simulink model "case2"  (R2024b)
settings: Solver=FixedStepAuto  StartTime=0  StopTime=1  FixedStep=1e-7  RelTol=1e-3
values from neighbouring files (symbols this model uses):
  SG_D_1_D = 0.01056    [IEEE9_case_parameters.m]    (also in case1_parameters.m; case2_parameters.m; case3_parameters.m; case4_parameters.m)
  SG_D_1_EnableSaturation = 0    [IEEE9_case_parameters.m]    (also in case1_parameters.m; case2_parameters.m; case3_parameters.m; case4_parameters.m)
  SG_D_1_f0 = 60    [IEEE9_case_parameters.m]    (also in case1_parameters.m; case2_parameters.m; case3_parameters.m; case4_parameters.m)
  SG_D_1_H = 7.5    [IEEE9_case_parameters.m]    (also in case1_parameters.m; case2_parameters.m; case3_parameters.m; case4_parameters.m)
  SG_D_1_K_A = 20    [IEEE9_case_parameters.m]    (also in case1_parameters.m; case2_parameters.m; case3_parameters.m; case4_parameters.m)
  SG_D_1_K_E = 1.000000e+1    (= 10)    [IEEE9_case_parameters.m]    (also in case1_parameters.m; case2_parameters.m; case3_parameters.m; case4_parameters.m)
  SG_D_1_K_F = 2.363    [IEEE9_case_parameters.m]    (also in case1_parameters.m; case2_parameters.m; case3_parameters.m; case4_parameters.m)
  SG_D_1_K_s = 0.5    [IEEE9_case_parameters.m]    (also in case1_parameters.m = 5; case2_parameters.m = 5; case3_parameters.m = 5; case4_parameters.m = 5)
  SG_D_1_R_a = 0.001088    [IEEE9_case_parameters.m]    (also in case1_parameters.m; case2_parameters.m; case3_parameters.m; case4_parameters.m)
  SG_D_1_S_A = 1    [IEEE9_case_parameters.m]    (also in case1_parameters.m; case2_parameters.m; case3_parameters.m; case4_parameters.m)
  SG_D_1_S_B = 0.103    [IEEE9_case_parameters.m]    (also in case1_parameters.m; case2_parameters.m; case3_parameters.m; case4_parameters.m)
  SG_D_1_S_N = 10.659857    [IEEE9_case_parameters.m]    (also in case1_parameters.m; case2_parameters.m; case3_parameters.m; case4_parameters.m)
  SG_D_1_SpeedPara = 200    [IEEE9_case_parameters.m]    (also in case1_parameters.m; case2_parameters.m; case3_parameters.m; case4_parameters.m)
  SG_D_1_T_0 = 0.720173    [IEEE9_case_parameters.m]    (also in case1_parameters.m = 0.755522; case2_parameters.m = 0.808931; case3_parameters.m = 0.869402; case4_parameters.m = 0.729316)
  SG_D_1_T_1 = 0.3    [IEEE9_case_parameters.m]    (also in case1_parameters.m; case2_parameters.m; case3_parameters.m; case4_parameters.m)
  SG_D_1_T_2 = 0.05    [IEEE9_case_parameters.m]    (also in case1_parameters.m; case2_parameters.m; case3_parameters.m; case4_parameters.m)
  SG_D_1_T_3 = 0.02    [IEEE9_case_parameters.m]    (also in case1_parameters.m; case2_parameters.m; case3_parameters.m; case4_parameters.m)
  SG_D_1_T_4 = 0.005    [IEEE9_case_parameters.m]    (also in case1_parameters.m; case2_parameters.m; case3_parameters.m; case4_parameters.m)
  SG_D_1_T_A = 0.02    [IEEE9_case_parameters.m]    (also in case1_parameters.m; case2_parameters.m; case3_parameters.m; case4_parameters.m)
  SG_D_1_T_dd = 8.000000e+0    (= 8)    [IEEE9_case_parameters.m]    (also in case1_parameters.m; case2_parameters.m; case3_parameters.m; case4_parameters.m)
  SG_D_1_T_ddd = 0.04    [IEEE9_case_parameters.m]    (also in case1_parameters.m; case2_parameters.m; case3_parameters.m; case4_parameters.m)
  SG_D_1_T_E = 0.314    [IEEE9_case_parameters.m]    (also in case1_parameters.m; case2_parameters.m; case3_parameters.m; case4_parameters.m)
  SG_D_1_T_F = 0.35    [IEEE9_case_parameters.m]    (also in case1_parameters.m; case2_parameters.m; case3_parameters.m; case4_parameters.m)
  SG_D_1_T_qd = 0.8    [IEEE9_case_parameters.m]    (also in case1_parameters.m; case2_parameters.m; case3_parameters.m; case4_parameters.m)
  SG_D_1_T_qdd = 0.02    [IEEE9_case_parameters.m]    (also in case1_parameters.m; case2_parameters.m; case3_parameters.m; case4_parameters.m)
  SG_D_1_T_speed = 0.1    [IEEE9_case_parameters.m]    (also in case1_parameters.m = 200; case2_parameters.m = 200; case3_parameters.m = 200; case4_parameters.m = 200)
  SG_D_1_T_w = 0.5    [IEEE9_case_parameters.m]    (also in case1_parameters.m; case2_parameters.m; case3_parameters.m; case4_parameters.m)
  SG_D_1_V_ref = 1.990276    [IEEE9_case_parameters.m]    (also in case1_parameters.m = 2.042296; case2_parameters.m = 2.051388; case3_parameters.m = 2.089584; case4_parameters.m = 2.01845)
  SG_D_1_w_ref = 376.991118    [IEEE9_case_parameters.m]    (also in case1_parameters.m; case2_parameters.m; case3_parameters.m; case4_parameters.m)
  SG_D_1_wb = 6.000000e+1    (= 60)    [IEEE9_case_parameters.m]    (also in case1_parameters.m; case2_parameters.m; case3_parameters.m; case4_parameters.m)
  SG_D_1_x_d = 1.9    [IEEE9_case_parameters.m]    (also in case1_parameters.m; case2_parameters.m; case3_parameters.m; case4_parameters.m)
  SG_D_1_x_dd = 0.302    [IEEE9_case_parameters.m]    (also in case1_parameters.m; case2_parameters.m; case3_parameters.m; case4_parameters.m)
  SG_D_1_x_ddd = 0.204    [IEEE9_case_parameters.m]    (also in case1_parameters.m; case2_parameters.m; case3_parameters.m; case4_parameters.m)
  SG_D_1_x_l = 0.05    [IEEE9_case_parameters.m]    (also in case1_parameters.m; case2_parameters.m; case3_parameters.m; case4_parameters.m)
  SG_D_1_x_q = 1.3    [IEEE9_case_parameters.m]    (also in case1_parameters.m; case2_parameters.m; case3_parameters.m; case4_parameters.m)
  SG_D_1_x_qd = 0.5    [IEEE9_case_parameters.m]    (also in case1_parameters.m; case2_parameters.m; case3_parameters.m; case4_parameters.m)
  SG_D_1_x_qdd = 0.3    [IEEE9_case_parameters.m]    (also in case1_parameters.m; case2_parameters.m; case3_parameters.m; case4_parameters.m)
  SG_D_2_D = 0.02    [IEEE9_case_parameters.m]    (also in case1_parameters.m; case2_parameters.m; case3_parameters.m; case4_parameters.m)
  SG_D_2_EnableSaturation = 0    [IEEE9_case_parameters.m]    (also in case1_parameters.m; case2_parameters.m; case3_parameters.m; case4_parameters.m)
  SG_D_2_f0 = 60    [IEEE9_case_parameters.m]    (also in case1_parameters.m; case2_parameters.m; case3_parameters.m; case4_parameters.m)
  SG_D_2_H = 8.000000e+0    (= 8)    [IEEE9_case_parameters.m]    (also in case1_parameters.m; case2_parameters.m; case3_parameters.m; case4_parameters.m)
  SG_D_2_K_A = 20    [IEEE9_case_parameters.m]    (also in case1_parameters.m; case2_parameters.m; case3_parameters.m; case4_parameters.m)
  SG_D_2_K_E = 1.000000e+1    (= 10)    [IEEE9_case_parameters.m]    (also in case1_parameters.m; case2_parameters.m; case3_parameters.m; case4_parameters.m)
  SG_D_2_K_F = 2.363    [IEEE9_case_parameters.m]    (also in case1_parameters.m; case2_parameters.m; case3_parameters.m; case4_parameters.m)
  SG_D_2_K_s = 0.5    [IEEE9_case_parameters.m]    (also in case1_parameters.m = 4; case2_parameters.m = 4; case3_parameters.m = 4; case4_parameters.m = 4)
  SG_D_2_R_a = 0.001088    [IEEE9_case_parameters.m]    (also in case1_parameters.m; case2_parameters.m; case3_parameters.m; case4_parameters.m)
  SG_D_2_S_A = 1    [IEEE9_case_parameters.m]    (also in case1_parameters.m; case2_parameters.m; case3_parameters.m; case4_parameters.m)
  SG_D_2_S_B = 0.103    [IEEE9_case_parameters.m]    (also in case1_parameters.m; case2_parameters.m; case3_parameters.m; case4_parameters.m)
  SG_D_2_S_N = 10.659857    [IEEE9_case_parameters.m]    (also in case1_parameters.m; case2_parameters.m; case3_parameters.m; case4_parameters.m)
  SG_D_2_SpeedPara = 200    [IEEE9_case_parameters.m]    (also in case1_parameters.m; case2_parameters.m; case3_parameters.m; case4_parameters.m)
  SG_D_2_T_0 = 1.632913    [IEEE9_case_parameters.m]    (also in case1_parameters.m = 1.632925; case2_parameters.m = 1.632915; case3_parameters.m = 1.632914; case4_parameters.m = 1.632927)
  SG_D_2_T_1 = 0.2    [IEEE9_case_parameters.m]    (also in case1_parameters.m; case2_parameters.m; case3_parameters.m; case4_parameters.m)
  SG_D_2_T_2 = 0.05    [IEEE9_case_parameters.m]    (also in case1_parameters.m; case2_parameters.m; case3_parameters.m; case4_parameters.m)
  SG_D_2_T_3 = 0.02    [IEEE9_case_parameters.m]    (also in case1_parameters.m; case2_parameters.m; case3_parameters.m; case4_parameters.m)
  SG_D_2_T_4 = 0.005    [IEEE9_case_parameters.m]    (also in case1_parameters.m; case2_parameters.m; case3_parameters.m; case4_parameters.m)
  SG_D_2_T_A = 0.02    [IEEE9_case_parameters.m]    (also in case1_parameters.m; case2_parameters.m; case3_parameters.m; case4_parameters.m)
  SG_D_2_T_dd = 7.9    [IEEE9_case_parameters.m]    (also in case1_parameters.m; case2_parameters.m; case3_parameters.m; case4_parameters.m)
  SG_D_2_T_ddd = 0.04    [IEEE9_case_parameters.m]    (also in case1_parameters.m; case2_parameters.m; case3_parameters.m; case4_parameters.m)
  SG_D_2_T_E = 0.314    [IEEE9_case_parameters.m]    (also in case1_parameters.m; case2_parameters.m; case3_parameters.m; case4_parameters.m)
  SG_D_2_T_F = 0.35    [IEEE9_case_parameters.m]    (also in case1_parameters.m; case2_parameters.m; case3_parameters.m; case4_parameters.m)
  SG_D_2_T_qd = 0.8    [IEEE9_case_parameters.m]    (also in case1_parameters.m; case2_parameters.m; case3_parameters.m; case4_parameters.m)
  SG_D_2_T_qdd = 0.015    [IEEE9_case_parameters.m]    (also in case1_parameters.m; case2_parameters.m; case3_parameters.m; case4_parameters.m)
  SG_D_2_T_speed = 0.1    [IEEE9_case_parameters.m]    (also in case1_parameters.m = 150; case2_parameters.m = 150; case3_parameters.m = 150; case4_parameters.m = 150)
  SG_D_2_T_w = 0.35    [IEEE9_case_parameters.m]    (also in case1_parameters.m; case2_parameters.m; case3_parameters.m; case4_parameters.m)
  SG_D_2_V_ref = 2.58547    [IEEE9_case_parameters.m]    (also in case1_parameters.m = 2.597896; case2_parameters.m = 2.587136; case3_parameters.m = 2.586042; case4_parameters.m = 2.599679)
  SG_D_2_w_ref = 376.991118    [IEEE9_case_parameters.m]    (also in case1_parameters.m; case2_parameters.m; case3_parameters.m; case4_parameters.m)
  SG_D_2_wb = 6.000000e+1    (= 60)    [IEEE9_case_parameters.m]    (also in case1_parameters.m; case2_parameters.m; case3_parameters.m; case4_parameters.m)
  SG_D_2_x_d = 1.8    [IEEE9_case_parameters.m]    (also in case1_parameters.m; case2_parameters.m; case3_parameters.m; case4_parameters.m)
  SG_D_2_x_dd = 0.302    [IEEE9_case_parameters.m]    (also in case1_parameters.m; case2_parameters.m; case3_parameters.m; case4_parameters.m)
  SG_D_2_x_ddd = 0.204    [IEEE9_case_parameters.m]    (also in case1_parameters.m; case2_parameters.m; case3_parameters.m; case4_parameters.m)
  SG_D_2_x_l = 0.05    [IEEE9_case_parameters.m]    (also in case1_parameters.m; case2_parameters.m; case3_parameters.m; case4_parameters.m)
  SG_D_2_x_q = 1.25    [IEEE9_case_parameters.m]    (also in case1_parameters.m; case2_parameters.m; case3_parameters.m; case4_parameters.m)
  SG_D_2_x_qd = 0.5    [IEEE9_case_parameters.m]    (also in case1_parameters.m; case2_parameters.m; case3_parameters.m; case4_parameters.m)
  SG_D_2_x_qdd = 0.3    [IEEE9_case_parameters.m]    (also in case1_parameters.m; case2_parameters.m; case3_parameters.m; case4_parameters.m)
  SG_D_3_D = 0.02    [IEEE9_case_parameters.m]    (also in case1_parameters.m; case2_parameters.m; case3_parameters.m; case4_parameters.m)
  SG_D_3_EnableSaturation = 0    [IEEE9_case_parameters.m]    (also in case1_parameters.m; case2_parameters.m; case3_parameters.m; case4_parameters.m)
  SG_D_3_f0 = 60    [IEEE9_case_parameters.m]    (also in case1_parameters.m; case2_parameters.m; case3_parameters.m; case4_parameters.m)
  SG_D_3_H = 7.7    [IEEE9_case_parameters.m]    (also in case1_parameters.m; case2_parameters.m; case3_parameters.m; case4_parameters.m)
  SG_D_3_K_A = 20    [IEEE9_case_parameters.m]    (also in case1_parameters.m; case2_parameters.m; case3_parameters.m; case4_parameters.m)
  SG_D_3_K_E = 1.000000e+1    (= 10)    [IEEE9_case_parameters.m]    (also in case1_parameters.m; case2_parameters.m; case3_parameters.m; case4_parameters.m)
  SG_D_3_K_F = 2.363    [IEEE9_case_parameters.m]    (also in case1_parameters.m; case2_parameters.m; case3_parameters.m; case4_parameters.m)
  SG_D_3_K_s = 0.2    [IEEE9_case_parameters.m]    (also in case1_parameters.m = 2; case2_parameters.m = 2; case3_parameters.m = 2; case4_parameters.m = 2)
  SG_D_3_R_a = 0.001088    [IEEE9_case_parameters.m]    (also in case1_parameters.m; case2_parameters.m; case3_parameters.m; case4_parameters.m)
  SG_D_3_S_A = 1    [IEEE9_case_parameters.m]    (also in case1_parameters.m; case2_parameters.m; case3_parameters.m; case4_parameters.m)
  SG_D_3_S_B = 0.103    [IEEE9_case_parameters.m]    (also in case1_parameters.m; case2_parameters.m; case3_parameters.m; case4_parameters.m)
  SG_D_3_S_N = 10.659857    [IEEE9_case_parameters.m]    (also in case1_parameters.m; case2_parameters.m; case3_parameters.m; case4_parameters.m)
  SG_D_3_SpeedPara = 200    [IEEE9_case_parameters.m]    (also in case1_parameters.m; case2_parameters.m; case3_parameters.m; case4_parameters.m)
  SG_D_3_T_0 = 0.850788    [IEEE9_case_parameters.m]    (also in case1_parameters.m = 0.850786; case2_parameters.m = 0.850787; case3_parameters.m; case4_parameters.m = 0.850786)
  SG_D_3_T_1 = 0.2    [IEEE9_case_parameters.m]    (also in case1_parameters.m; case2_parameters.m; case3_parameters.m; case4_parameters.m)
  SG_D_3_T_2 = 0.05    [IEEE9_case_parameters.m]    (also in case1_parameters.m; case2_parameters.m; case3_parameters.m; case4_parameters.m)
  SG_D_3_T_3 = 0.02    [IEEE9_case_parameters.m]    (also in case1_parameters.m; case2_parameters.m; case3_parameters.m; case4_parameters.m)
  SG_D_3_T_4 = 0.005    [IEEE9_case_parameters.m]    (also in case1_parameters.m; case2_parameters.m; case3_parameters.m; case4_parameters.m)
  SG_D_3_T_A = 0.02    [IEEE9_case_parameters.m]    (also in case1_parameters.m; case2_parameters.m; case3_parameters.m; case4_parameters.m)
  SG_D_3_T_dd = 8.1    [IEEE9_case_parameters.m]    (also in case1_parameters.m; case2_parameters.m; case3_parameters.m; case4_parameters.m)
  SG_D_3_T_ddd = 0.04    [IEEE9_case_parameters.m]    (also in case1_parameters.m; case2_parameters.m; case3_parameters.m; case4_parameters.m)
  SG_D_3_T_E = 0.314    [IEEE9_case_parameters.m]    (also in case1_parameters.m; case2_parameters.m; case3_parameters.m; case4_parameters.m)
  SG_D_3_T_F = 0.35    [IEEE9_case_parameters.m]    (also in case1_parameters.m; case2_parameters.m; case3_parameters.m; case4_parameters.m)
  SG_D_3_T_qd = 0.8    [IEEE9_case_parameters.m]    (also in case1_parameters.m; case2_parameters.m; case3_parameters.m; case4_parameters.m)
  SG_D_3_T_qdd = 0.015    [IEEE9_case_parameters.m]    (also in case1_parameters.m; case2_parameters.m; case3_parameters.m; case4_parameters.m)
  SG_D_3_T_speed = 0.1    [IEEE9_case_parameters.m]    (also in case1_parameters.m = 180; case2_parameters.m = 180; case3_parameters.m = 180; case4_parameters.m = 180)
  SG_D_3_T_w = 0.4    [IEEE9_case_parameters.m]    (also in case1_parameters.m; case2_parameters.m; case3_parameters.m; case4_parameters.m)
  SG_D_3_V_ref = 1.892727    [IEEE9_case_parameters.m]    (also in case1_parameters.m = 1.906439; case2_parameters.m = 1.895535; case3_parameters.m = 1.892105; case4_parameters.m = 1.906598)
  SG_D_3_w_ref = 376.991118    [IEEE9_case_parameters.m]    (also in case1_parameters.m; case2_parameters.m; case3_parameters.m; case4_parameters.m)
  SG_D_3_wb = 6.000000e+1    (= 60)    [IEEE9_case_parameters.m]    (also in case1_parameters.m; case2_parameters.m; case3_parameters.m; case4_parameters.m)
  SG_D_3_x_d = 1.85    [IEEE9_case_parameters.m]    (also in case1_parameters.m; case2_parameters.m; case3_parameters.m; case4_parameters.m)
  SG_D_3_x_dd = 0.302    [IEEE9_case_parameters.m]    (also in case1_parameters.m; case2_parameters.m; case3_parameters.m; case4_parameters.m)
  SG_D_3_x_ddd = 0.204    [IEEE9_case_parameters.m]    (also in case1_parameters.m; case2_parameters.m; case3_parameters.m; case4_parameters.m)
  SG_D_3_x_l = 0.05    [IEEE9_case_parameters.m]    (also in case1_parameters.m; case2_parameters.m; case3_parameters.m; case4_parameters.m)
  SG_D_3_x_q = 1.2    [IEEE9_case_parameters.m]    (also in case1_parameters.m; case2_parameters.m; case3_parameters.m; case4_parameters.m)
  SG_D_3_x_qd = 0.5    [IEEE9_case_parameters.m]    (also in case1_parameters.m; case2_parameters.m; case3_parameters.m; case4_parameters.m)
  SG_D_3_x_qdd = 0.3    [IEEE9_case_parameters.m]    (also in case1_parameters.m; case2_parameters.m; case3_parameters.m; case4_parameters.m)
(part 4 of 12)

== system case2/AC_1/d_vq_bus_7_block ==
  note: d_vq_bus_7 in case2
      | $2106.09563369148\,\mathrm{iq}_{\mathrm{bus},7}-376.991118430775\,\mathrm{vd}_{\mathrm{bus},7}$
      | Automatically generated on 2025-10-31 18:56:40 .
  Alge_iq_bus_7_7a913 : Inport
  State_vd_bus_7_25da7 : Inport  Port=2
  Constant_2106.09563369148_6eec0 : Constant  Value=2106.09563369148
  Constant_376.991118430775_6db8e : Constant  Value=376.991118430775
  Product_2c008 : Product
  Product_e182c : Product
  Subtract_8240b : Sum  Inputs=+-
  Blockout_d_vq_bus_7_d417b : Outport
  wires:
  Constant_2106.09563369148_6eec0/1 -> Product_e182c/1
  Product_2c008/1 -> Subtract_8240b/2
  Alge_iq_bus_7_7a913/1 -> Product_e182c/2
  Constant_376.991118430775_6db8e/1 -> Product_2c008/1
  Subtract_8240b/1 -> Blockout_d_vq_bus_7_d417b/1
  State_vd_bus_7_25da7/1 -> Product_2c008/2
  Product_e182c/1 -> Subtract_8240b/1

== system case2/AC_1/d_vq_bus_8_block ==
  note: d_vq_bus_8 in case2
      | $1657.10381727813\,\mathrm{iq}_{\mathrm{bus},8}-376.991118430775\,\mathrm{vd}_{\mathrm{bus},8}$
      | Automatically generated on 2025-10-31 18:56:41 .
  Alge_iq_bus_8_0994e : Inport
  State_vd_bus_8_fb157 : Inport  Port=2
  Constant_1657.10381727813_190e7 : Constant  Value=1657.10381727813
  Constant_376.991118430775_a2048 : Constant  Value=376.991118430775
  Product_78e61 : Product
  Product_91dd3 : Product
  Subtract_5bb88 : Sum  Inputs=+-
  Blockout_d_vq_bus_8_66a55 : Outport
  wires:
  Constant_1657.10381727813_190e7/1 -> Product_78e61/1
  Constant_376.991118430775_a2048/1 -> Product_91dd3/1
  Alge_iq_bus_8_0994e/1 -> Product_78e61/2
  State_vd_bus_8_fb157/1 -> Product_91dd3/2
  Product_78e61/1 -> Subtract_5bb88/1
  Product_91dd3/1 -> Subtract_5bb88/2
  Subtract_5bb88/1 -> Blockout_d_vq_bus_8_66a55/1

== system case2/AC_1/d_vq_bus_9_block ==
  note: d_vq_bus_9 in case2
      | $1564.27849971276\,\mathrm{iq}_{\mathrm{bus},9}-376.991118430775\,\mathrm{vd}_{\mathrm{bus},9}$
      | Automatically generated on 2025-10-31 18:56:43 .
  Alge_iq_bus_9_5bc50 : Inport
  State_vd_bus_9_96e3e : Inport  Port=2
  Constant_1564.27849971276_94c7c : Constant  Value=1564.27849971276
  Constant_376.991118430775_75168 : Constant  Value=376.991118430775
  Product_63ca6 : Product
  Product_a286d : Product
  Subtract_c7145 : Sum  Inputs=+-
  Blockout_d_vq_bus_9_3fd84 : Outport
  wires:
  Constant_1564.27849971276_94c7c/1 -> Product_a286d/1
  Constant_376.991118430775_75168/1 -> Product_63ca6/1
  Alge_iq_bus_9_5bc50/1 -> Product_a286d/2
  State_vd_bus_9_96e3e/1 -> Product_63ca6/2
  Product_a286d/1 -> Subtract_c7145/1
  Product_63ca6/1 -> Subtract_c7145/2
  Subtract_c7145/1 -> Blockout_d_vq_bus_9_3fd84/1

== system case2/AC_1/id_bus_1_block ==
  note: id_bus_1 in case2
      | $\mathrm{id}_{\mathrm{SG},D,1}-\mathrm{id}_{\mathrm{line},1,4}$
      | Automatically generated on 2025-10-31 18:57:12 .
  Input_id_SG_D_1_a599e : Inport
  State_id_line_1_4_e0f83 : Inport  Port=2
  Subtract_3836a : Sum  Inputs=+-
  Blockout_id_bus_1_49cc3 : Outport
  wires:
  Input_id_SG_D_1_a599e/1 -> Subtract_3836a/1
  State_id_line_1_4_e0f83/1 -> Subtract_3836a/2
  Subtract_3836a/1 -> Blockout_id_bus_1_49cc3/1

== system case2/AC_1/id_bus_2_block ==
  note: id_bus_2 in case2
      | $\mathrm{id}_{\mathrm{SG},D,2}+\mathrm{id}_{\mathrm{line},8,2}$
      | Automatically generated on 2025-10-31 18:57:14 .
  Input_id_SG_D_2_544c5 : Inport
  State_id_line_8_2_af6d6 : Inport  Port=2
  Add_25965 : Sum
  Blockout_id_bus_2_a8585 : Outport
  wires:
  Input_id_SG_D_2_544c5/1 -> Add_25965/1
  State_id_line_8_2_af6d6/1 -> Add_25965/2
  Add_25965/1 -> Blockout_id_bus_2_a8585/1

== system case2/AC_1/id_bus_3_block ==
  note: id_bus_3 in case2
      | $\mathrm{id}_{\mathrm{SG},D,3}-\mathrm{id}_{\mathrm{line},3,6}$
      | Automatically generated on 2025-10-31 18:57:17 .
  Input_id_SG_D_3_1b557 : Inport
  State_id_line_3_6_b321d : Inport  Port=2
  Subtract_b0912 : Sum  Inputs=+-
  Blockout_id_bus_3_1118d : Outport
  wires:
  Input_id_SG_D_3_1b557/1 -> Subtract_b0912/1
  State_id_line_3_6_b321d/1 -> Subtract_b0912/2
  Subtract_b0912/1 -> Blockout_id_bus_3_1118d/1

== system case2/AC_1/id_bus_4_block ==
  note: id_bus_4 in case2
      | $\mathrm{id}_{\mathrm{line},1,4}-\mathrm{id}_{\mathrm{line},4,5}+\mathrm{id}_{\mathrm{line},9,4}$
      | Automatically generated on 2025-10-31 18:57:18 .
  State_id_line_1_4_2b5ff : Inport
  State_id_line_4_5_50091 : Inport  Port=2
  State_id_line_9_4_0046a : Inport  Port=3
  Add_47ed8 : Sum
  Subtract_ce8ae : Sum  Inputs=+-
  Blockout_id_bus_4_748d0 : Outport
  wires:
  State_id_line_9_4_0046a/1 -> Add_47ed8/2
  State_id_line_1_4_2b5ff/1 -> Subtract_ce8ae/1
  State_id_line_4_5_50091/1 -> Subtract_ce8ae/2
  Subtract_ce8ae/1 -> Add_47ed8/1
  Add_47ed8/1 -> Blockout_id_bus_4_748d0/1

== system case2/AC_1/id_bus_5_block ==
  note: id_bus_5 in case2
      | $\mathrm{id}_{\mathrm{line},4,5}-\mathrm{id}_{\mathrm{load},5}-\mathrm{id}_{\mathrm{line},5,6}$
      | Automatically generated on 2025-10-31 18:57:19 .
  State_id_load_5_a31e5 : Inport
  State_id_line_4_5_6f8c4 : Inport  Port=2
  State_id_line_5_6_04a55 : Inport  Port=3
  Add_06c24 : Sum
  Constant_-1_18fea : Constant  Value=-1
  Product_bc2c4 : Product
  Subtract_dde7b : Sum  Inputs=+-
  Blockout_id_bus_5_7e5b8 : Outport
  wires:
  Subtract_dde7b/1 -> Blockout_id_bus_5_7e5b8/1
  State_id_line_4_5_6f8c4/1 -> Add_06c24/2
  Constant_-1_18fea/1 -> Product_bc2c4/1
  Add_06c24/1 -> Subtract_dde7b/1
  State_id_load_5_a31e5/1 -> Product_bc2c4/2
  Product_bc2c4/1 -> Add_06c24/1
  State_id_line_5_6_04a55/1 -> Subtract_dde7b/2

== system case2/AC_1/id_bus_6_block ==
  note: id_bus_6 in case2
      | $\mathrm{id}_{\mathrm{line},3,6}+\mathrm{id}_{\mathrm{line},5,6}-\mathrm{id}_{\mathrm{line},6,7}$
      | Automatically generated on 2025-10-31 18:57:21 .
  State_id_line_3_6_3a667 : Inport
  State_id_line_5_6_c534c : Inport  Port=2
  State_id_line_6_7_02fca : Inport  Port=3
  Add_621a3 : Sum
  Subtract_b574d : Sum  Inputs=+-
  Blockout_id_bus_6_b1df2 : Outport
  wires:
  State_id_line_6_7_02fca/1 -> Subtract_b574d/2
  State_id_line_3_6_3a667/1 -> Add_621a3/1
  State_id_line_5_6_c534c/1 -> Add_621a3/2
  Add_621a3/1 -> Subtract_b574d/1
  Subtract_b574d/1 -> Blockout_id_bus_6_b1df2/1

== system case2/AC_1/id_bus_7_block ==
  note: id_bus_7 in case2
      | $\mathrm{id}_{\mathrm{line},6,7}-\mathrm{id}_{\mathrm{load},7}-\mathrm{id}_{\mathrm{line},7,8}$
      | Automatically generated on 2025-10-31 18:57:22 .
  State_id_load_7_161b2 : Inport
  State_id_line_6_7_c74f6 : Inport  Port=2
  State_id_line_7_8_561bd : Inport  Port=3
  Add_fd93d : Sum
  Constant_-1_8de6e : Constant  Value=-1
  Product_509df : Product
  Subtract_5c369 : Sum  Inputs=+-
  Blockout_id_bus_7_4fd6a : Outport
  wires:
  Subtract_5c369/1 -> Blockout_id_bus_7_4fd6a/1
  State_id_line_6_7_c74f6/1 -> Add_fd93d/2
  Constant_-1_8de6e/1 -> Product_509df/1
  Add_fd93d/1 -> Subtract_5c369/1
  State_id_load_7_161b2/1 -> Product_509df/2
  Product_509df/1 -> Add_fd93d/1
  State_id_line_7_8_561bd/1 -> Subtract_5c369/2

== system case2/AC_1/id_bus_8_block ==
  note: id_bus_8 in case2
      | $\mathrm{id}_{\mathrm{line},7,8}-\mathrm{id}_{\mathrm{line},8,2}-\mathrm{id}_{\mathrm{line},8,9}$
      | Automatically generated on 2025-10-31 18:57:24 .
  State_id_line_7_8_11373 : Inport
  State_id_line_8_2_95418 : Inport  Port=2
  State_id_line_8_9_a20e3 : Inport  Port=3
  Subtract_b826c : Sum  Inputs=+-
  Subtract_ed5db : Sum  Inputs=+-
  Blockout_id_bus_8_d4ccc : Outport
  wires:
  State_id_line_8_9_a20e3/1 -> Subtract_b826c/2
  State_id_line_7_8_11373/1 -> Subtract_ed5db/1
  State_id_line_8_2_95418/1 -> Subtract_ed5db/2
  Subtract_ed5db/1 -> Subtract_b826c/1
  Subtract_b826c/1 -> Blockout_id_bus_8_d4ccc/1

== system case2/AC_1/id_bus_9_block ==
  note: id_bus_9 in case2
      | $\mathrm{id}_{\mathrm{line},8,9}-\mathrm{id}_{\mathrm{load},9}-\mathrm{id}_{\mathrm{line},9,4}$
      | Automatically generated on 2025-10-31 18:57:25 .
  State_id_load_9_97526 : Inport
  State_id_line_8_9_07115 : Inport  Port=2
  State_id_line_9_4_b960f : Inport  Port=3
  Add_9c2ef : Sum
  Constant_-1_d81ed : Constant  Value=-1
  Product_e3bb5 : Product
  Subtract_dd3f4 : Sum  Inputs=+-
  Blockout_id_bus_9_2e79f : Outport
  wires:
  Subtract_dd3f4/1 -> Blockout_id_bus_9_2e79f/1
  State_id_line_8_9_07115/1 -> Add_9c2ef/2
  Constant_-1_d81ed/1 -> Product_e3bb5/1
  Add_9c2ef/1 -> Subtract_dd3f4/1
  State_id_load_9_97526/1 -> Product_e3bb5/2
  Product_e3bb5/1 -> Add_9c2ef/1
  State_id_line_9_4_b960f/1 -> Subtract_dd3f4/2

== system case2/AC_1/iq_bus_1_block ==
  note: iq_bus_1 in case2
      | $\mathrm{iq}_{\mathrm{SG},D,1}-\mathrm{iq}_{\mathrm{line},1,4}$
      | Automatically generated on 2025-10-31 18:57:13 .
  Input_iq_SG_D_1_56b6f : Inport
  State_iq_line_1_4_7b28f : Inport  Port=2
  Subtract_6d19f : Sum  Inputs=+-
  Blockout_iq_bus_1_79d62 : Outport
  wires:
  Input_iq_SG_D_1_56b6f/1 -> Subtract_6d19f/1
  State_iq_line_1_4_7b28f/1 -> Subtract_6d19f/2
  Subtract_6d19f/1 -> Blockout_iq_bus_1_79d62/1

== system case2/AC_1/iq_bus_2_block ==
  note: iq_bus_2 in case2
      | $\mathrm{iq}_{\mathrm{SG},D,2}+\mathrm{iq}_{\mathrm{line},8,2}$
      | Automatically generated on 2025-10-31 18:57:15 .
  Input_iq_SG_D_2_708e6 : Inport
  State_iq_line_8_2_8ad2f : Inport  Port=2
  Add_3659d : Sum
  Blockout_iq_bus_2_b5069 : Outport
  wires:
  Input_iq_SG_D_2_708e6/1 -> Add_3659d/1
  State_iq_line_8_2_8ad2f/1 -> Add_3659d/2
  Add_3659d/1 -> Blockout_iq_bus_2_b5069/1

== system case2/AC_1/iq_bus_3_block ==
  note: iq_bus_3 in case2
      | $\mathrm{iq}_{\mathrm{SG},D,3}-\mathrm{iq}_{\mathrm{line},3,6}$
      | Automatically generated on 2025-10-31 18:57:17 .
  Input_iq_SG_D_3_22043 : Inport
  State_iq_line_3_6_4d41b : Inport  Port=2
  Subtract_f9fe4 : Sum  Inputs=+-
  Blockout_iq_bus_3_7dfe9 : Outport
  wires:
  Input_iq_SG_D_3_22043/1 -> Subtract_f9fe4/1
  State_iq_line_3_6_4d41b/1 -> Subtract_f9fe4/2
  Subtract_f9fe4/1 -> Blockout_iq_bus_3_7dfe9/1

== system case2/AC_1/iq_bus_4_block ==
  note: iq_bus_4 in case2
      | $\mathrm{iq}_{\mathrm{line},1,4}-\mathrm{iq}_{\mathrm{line},4,5}+\mathrm{iq}_{\mathrm{line},9,4}$
      | Automatically generated on 2025-10-31 18:57:19 .
  State_iq_line_1_4_47e2e : Inport
  State_iq_line_4_5_efb88 : Inport  Port=2
  State_iq_line_9_4_15ad7 : Inport  Port=3
  Add_69af6 : Sum
  Subtract_6a82e : Sum  Inputs=+-
  Blockout_iq_bus_4_79ed0 : Outport
  wires:
  State_iq_line_1_4_47e2e/1 -> Subtract_6a82e/1
  State_iq_line_4_5_efb88/1 -> Subtract_6a82e/2
  Subtract_6a82e/1 -> Add_69af6/1
  State_iq_line_9_4_15ad7/1 -> Add_69af6/2
  Add_69af6/1 -> Blockout_iq_bus_4_79ed0/1

== system case2/AC_1/iq_bus_5_block ==
  note: iq_bus_5 in case2
      | $\mathrm{iq}_{\mathrm{line},4,5}-\mathrm{iq}_{\mathrm{load},5}-\mathrm{iq}_{\mathrm{line},5,6}$
      | Automatically generated on 2025-10-31 18:57:20 .
  State_iq_load_5_a6c3f : Inport
  State_iq_line_4_5_553d2 : Inport  Port=2
  State_iq_line_5_6_211b7 : Inport  Port=3
  Add_5a667 : Sum
  Constant_-1_5bc1c : Constant  Value=-1
  Product_5bf4b : Product
  Subtract_c2b7f : Sum  Inputs=+-
  Blockout_iq_bus_5_9f39d : Outport
  wires:
  Subtract_c2b7f/1 -> Blockout_iq_bus_5_9f39d/1
  State_iq_line_4_5_553d2/1 -> Add_5a667/2
  Constant_-1_5bc1c/1 -> Product_5bf4b/1
  State_iq_load_5_a6c3f/1 -> Product_5bf4b/2
  Product_5bf4b/1 -> Add_5a667/1
  Add_5a667/1 -> Subtract_c2b7f/1
  State_iq_line_5_6_211b7/1 -> Subtract_c2b7f/2

== system case2/AC_1/iq_bus_6_block ==
  note: iq_bus_6 in case2
      | $\mathrm{iq}_{\mathrm{line},3,6}+\mathrm{iq}_{\mathrm{line},5,6}-\mathrm{iq}_{\mathrm{line},6,7}$
      | Automatically generated on 2025-10-31 18:57:22 .
  State_iq_line_3_6_ec9b9 : Inport
  State_iq_line_5_6_6d34c : Inport  Port=2
  State_iq_line_6_7_450ec : Inport  Port=3
  Add_a6e35 : Sum
  Subtract_569d7 : Sum  Inputs=+-
  Blockout_iq_bus_6_d8605 : Outport
  wires:
  State_iq_line_3_6_ec9b9/1 -> Add_a6e35/1
  State_iq_line_5_6_6d34c/1 -> Add_a6e35/2
  Add_a6e35/1 -> Subtract_569d7/1
  State_iq_line_6_7_450ec/1 -> Subtract_569d7/2
  Subtract_569d7/1 -> Blockout_iq_bus_6_d8605/1

== system case2/AC_1/iq_bus_7_block ==
  note: iq_bus_7 in case2
      | $\mathrm{iq}_{\mathrm{line},6,7}-\mathrm{iq}_{\mathrm{load},7}-\mathrm{iq}_{\mathrm{line},7,8}$
      | Automatically generated on 2025-10-31 18:57:23 .
  State_iq_load_7_d4d4f : Inport
  State_iq_line_6_7_cab3a : Inport  Port=2
  State_iq_line_7_8_f10ed : Inport  Port=3
  Add_cdcfb : Sum
  Constant_-1_1c705 : Constant  Value=-1
  Product_95b8a : Product
  Subtract_ee63b : Sum  Inputs=+-
  Blockout_iq_bus_7_1b282 : Outport
  wires:
  Subtract_ee63b/1 -> Blockout_iq_bus_7_1b282/1
  State_iq_line_6_7_cab3a/1 -> Add_cdcfb/2
  Constant_-1_1c705/1 -> Product_95b8a/1
  State_iq_load_7_d4d4f/1 -> Product_95b8a/2
  Product_95b8a/1 -> Add_cdcfb/1
  Add_cdcfb/1 -> Subtract_ee63b/1
  State_iq_line_7_8_f10ed/1 -> Subtract_ee63b/2

== system case2/AC_1/iq_bus_8_block ==
  note: iq_bus_8 in case2
      | $\mathrm{iq}_{\mathrm{line},7,8}-\mathrm{iq}_{\mathrm{line},8,2}-\mathrm{iq}_{\mathrm{line},8,9}$
      | Automatically generated on 2025-10-31 18:57:25 .
  State_iq_line_7_8_0fde7 : Inport
  State_iq_line_8_2_e4d44 : Inport  Port=2
  State_iq_line_8_9_635a9 : Inport  Port=3
  Subtract_88351 : Sum  Inputs=+-
  Subtract_f737a : Sum  Inputs=+-
  Blockout_iq_bus_8_11109 : Outport
  wires:
  State_iq_line_7_8_0fde7/1 -> Subtract_f737a/1
  State_iq_line_8_2_e4d44/1 -> Subtract_f737a/2
  Subtract_f737a/1 -> Subtract_88351/1
  State_iq_line_8_9_635a9/1 -> Subtract_88351/2
  Subtract_88351/1 -> Blockout_iq_bus_8_11109/1

== system case2/AC_1/iq_bus_9_block ==
  note: iq_bus_9 in case2
      | $\mathrm{iq}_{\mathrm{line},8,9}-\mathrm{iq}_{\mathrm{load},9}-\mathrm{iq}_{\mathrm{line},9,4}$
      | Automatically generated on 2025-10-31 18:57:26 .
  State_iq_load_9_0a6dd : Inport
  State_iq_line_8_9_83b30 : Inport  Port=2
  State_iq_line_9_4_aebff : Inport  Port=3
  Add_b8fe7 : Sum
  Constant_-1_4a85c : Constant  Value=-1
  Product_b57fd : Product
  Subtract_a29b7 : Sum  Inputs=+-
  Blockout_iq_bus_9_46ecf : Outport
  wires:
  Subtract_a29b7/1 -> Blockout_iq_bus_9_46ecf/1
  State_iq_line_8_9_83b30/1 -> Add_b8fe7/2
  Constant_-1_4a85c/1 -> Product_b57fd/1
  State_iq_load_9_0a6dd/1 -> Product_b57fd/2
  Product_b57fd/1 -> Add_b8fe7/1
  Add_b8fe7/1 -> Subtract_a29b7/1
  State_iq_line_9_4_aebff/1 -> Subtract_a29b7/2

== system case2/AC_1/vd_bus_1_out_block ==
  note: vd_bus_1_out in case2
      | $\mathrm{vd}_{\mathrm{bus},1}$
      | Automatically generated on 2025-10-31 18:57:11 .
  State_vd_bus_1_5e32d : Inport
  Blockout_vd_bus_1_out_57e66 : Outport
  wires:
  State_vd_bus_1_5e32d/1 -> Blockout_vd_bus_1_out_57e66/1

== system case2/AC_1/vd_bus_2_out_block ==
  note: vd_bus_2_out in case2
      | $\mathrm{vd}_{\mathrm{bus},2}$
      | Automatically generated on 2025-10-31 18:57:13 .
  State_vd_bus_2_38fae : Inport
  Blockout_vd_bus_2_out_3230a : Outport
  wires:
  State_vd_bus_2_38fae/1 -> Blockout_vd_bus_2_out_3230a/1

== system case2/AC_1/vd_bus_3_out_block ==
  note: vd_bus_3_out in case2
      | $\mathrm{vd}_{\mathrm{bus},3}$
      | Automatically generated on 2025-10-31 18:57:16 .
  State_vd_bus_3_18f77 : Inport
  Blockout_vd_bus_3_out_24978 : Outport
  wires:
  State_vd_bus_3_18f77/1 -> Blockout_vd_bus_3_out_24978/1

== system case2/AC_1/vq_bus_1_out_block ==
  note: vq_bus_1_out in case2
      | $\mathrm{vq}_{\mathrm{bus},1}$
      | Automatically generated on 2025-10-31 18:57:11 .
  State_vq_bus_1_b3dd1 : Inport
  Blockout_vq_bus_1_out_5135a : Outport
  wires:
  State_vq_bus_1_b3dd1/1 -> Blockout_vq_bus_1_out_5135a/1

== system case2/AC_1/vq_bus_2_out_block ==
  note: vq_bus_2_out in case2
      | $\mathrm{vq}_{\mathrm{bus},2}$
      | Automatically generated on 2025-10-31 18:57:14 .
  State_vq_bus_2_b12fe : Inport
  Blockout_vq_bus_2_out_0c630 : Outport
  wires:
  State_vq_bus_2_b12fe/1 -> Blockout_vq_bus_2_out_0c630/1

== system case2/AC_1/vq_bus_3_out_block ==
  note: vq_bus_3_out in case2
      | $\mathrm{vq}_{\mathrm{bus},3}$
      | Automatically generated on 2025-10-31 18:57:16 .
  State_vq_bus_3_f0d02 : Inport
  Blockout_vq_bus_3_out_fc8db : Outport
  wires:
  State_vq_bus_3_f0d02/1 -> Blockout_vq_bus_3_out_fc8db/1

== system case2/SG_D_1/T_e_SG_D_1_block ==
  note: T_e_SG_D_1 in case2
      | $-\frac{\psi _{d,\mathrm{SG},D,1}\,\left(\psi _{q,\mathrm{SG},D,1}+\frac{\psi _{\mathrm{gq},\mathrm{SG},D,1}\,\left(x_{l}-x_{\mathrm{qdd}}\right)}{x_{l}-x_{\mathrm{qd}}}+\frac{\psi _{\mathrm{kq},\mathrm{SG},D,1}\,\left(x_{\mathrm{qd}}-x_{\mathrm{qdd}}\right)}{x_{l}-x_{\mathrm{qd}}}\right)}{x_{\mathrm{qdd}}}-\frac{\psi _{q,\mathrm{SG},D,1}\,\left(\frac{\psi _{\mathrm{1d},\mathrm{SG},D,1}\,\left(x_{\mathrm{dd}}-x_{\mathrm{ddd}}\right)}{x_{\mathrm{dd}}-x_{l}}-\psi _{d,\mathrm{SG},D,1}+\frac{\psi _{\mathrm{fd},\mathrm{SG},D,1}\,\left(x_{\mathrm{ddd}}-x_{l}\right)}{x_{\mathrm{dd}}-x_{l}}\right)}{x_{\mathrm{ddd}}}$
      | Automatically generated on 2025-10-31 18:53:59 .
  State_psi_d_SG_D_1_175f2 : Inport
  State_psi_gq_SG_D_1_90d07 : Inport  Port=2
  State_psi_kq_SG_D_1_d34b9 : Inport  Port=3
  State_psi_q_SG_D_1_e9ca1 : Inport  Port=4
  State_psi_q_SG_D_1_1eaa9 : Inport  Port=5
  State_psi_1d_SG_D_1_6b7a6 : Inport  Port=6
  State_psi_d_SG_D_1_deb78 : Inport  Port=7
  State_psi_fd_SG_D_1_72d5b : Inport  Port=8
  Add_0aa48 : Sum
  Add_340b6 : Sum
  Add_3d244 : Sum
  Add_4d303 : Sum
  Add_9a46d : Sum
  Add_bc191 : Sum
  Constant_-1_0f8c1 : Constant  Value=-1
  Constant_-1_170f2 : Constant  Value=-1
  Constant_-1_22821 : Constant  Value=-1
  Constant_-1_b75c6 : Constant  Value=-1
  Constant_-1_f97ae : Constant  Value=-1
  Constant_x_dd_3564b : Constant  Value=x_dd
  Constant_x_dd_a0dd6 : Constant  Value=x_dd
  Constant_x_dd_c6452 : Constant  Value=x_dd
  Constant_x_ddd_2cff1 : Constant  Value=x_ddd
  Constant_x_ddd_5dfba : Constant  Value=x_ddd
  Constant_x_ddd_b1933 : Constant  Value=x_ddd
  Constant_x_l_138de : Constant  Value=x_l
  Constant_x_l_921cd : Constant  Value=x_l
  Constant_x_l_acc66 : Constant  Value=x_l
  Constant_x_l_ad689 : Constant  Value=x_l
  Constant_x_l_b742d : Constant  Value=x_l
  Constant_x_l_ee615 : Constant  Value=x_l
  Constant_x_qd_445bc : Constant  Value=x_qd
  Constant_x_qd_48d6e : Constant  Value=x_qd
  Constant_x_qd_d85e7 : Constant  Value=x_qd
  Constant_x_qdd_07b7b : Constant  Value=x_qdd
  Constant_x_qdd_93d43 : Constant  Value=x_qdd
  Constant_x_qdd_c6d91 : Constant  Value=x_qdd
  Divide_01188 : Product  Inputs=*/
  Divide_30e86 : Product  Inputs=*/
  Divide_541d7 : Product  Inputs=*/
  Divide_61e29 : Product  Inputs=*/
  Divide_93cdc : Product  Inputs=*/
  Divide_ed81b : Product  Inputs=*/
  Product_1a907 : Product
  Product_25ba4 : Product
  Product_33a84 : Product
  Product_4d3cc : Product
  Product_698f7 : Product
  Product_ad06a : Product
  Product_babae : Product
  Product_c9689 : Product
  Product_ce255 : Product
  Product_f807f : Product
  Product_fabca : Product
  Subtract_1dd49 : Sum  Inputs=+-
  Subtract_20a40 : Sum  Inputs=+-
  Subtract_32e12 : Sum  Inputs=+-
  Subtract_54444 : Sum  Inputs=+-
  Subtract_5c8ce : Sum  Inputs=+-
  Subtract_aea2e : Sum  Inputs=+-
  Subtract_b8578 : Sum  Inputs=+-
  Blockout_T_e_SG_D_1_032d2 : Outport
  wires:
  Product_fabca/1 -> Divide_61e29/1
  Product_f807f/1 -> Add_9a46d/1
  Divide_61e29/1 -> Subtract_20a40/1
  Constant_-1_f97ae/1 -> Product_f807f/1
  Constant_x_l_138de/1 -> Product_f807f/2
  Constant_x_qdd_c6d91/1 -> Add_9a46d/2
  Constant_x_qd_445bc/1 -> Subtract_b8578/1
  Constant_-1_b75c6/1 -> Product_1a907/1
  Constant_x_qdd_07b7b/1 -> Divide_01188/2
  Constant_x_qdd_93d43/1 -> Subtract_b8578/2
  State_psi_q_SG_D_1_1eaa9/1 -> Product_25ba4/1
  Constant_x_dd_c6452/1 -> Subtract_5c8ce/1
  Constant_x_l_b742d/1 -> Product_1a907/2
  Subtract_5c8ce/1 -> Product_698f7/2
  Constant_-1_0f8c1/1 -> Product_33a84/1
  Constant_x_l_ad689/1 -> Product_33a84/2
  Subtract_aea2e/1 -> Product_25ba4/2
  State_psi_q_SG_D_1_e9ca1/1 -> Add_0aa48/2
  Constant_-1_22821/1 -> Product_ce255/1
  State_psi_1d_SG_D_1_6b7a6/1 -> Product_ce255/2
  Constant_x_ddd_5dfba/1 -> Subtract_5c8ce/2
  State_psi_gq_SG_D_1_90d07/1 -> Product_fabca/1
  Add_9a46d/1 -> Product_fabca/2
  Product_1a907/1 -> Add_3d244/1
  Product_ad06a/1 -> Product_4d3cc/1
  Constant_x_qd_d85e7/1 -> Add_3d244/2
  Product_698f7/1 -> Divide_30e86/1
  State_psi_kq_SG_D_1_d34b9/1 -> Product_c9689/1
  Add_3d244/1 -> Divide_61e29/2
  Subtract_b8578/1 -> Product_c9689/2
  Product_33a84/1 -> Add_bc191/1
  Constant_x_qd_48d6e/1 -> Add_bc191/2
  Product_c9689/1 -> Divide_93cdc/1
  Product_ce255/1 -> Product_698f7/1
  Constant_x_dd_a0dd6/1 -> Subtract_32e12/1
  Constant_x_l_ee615/1 -> Subtract_32e12/2
  Constant_x_ddd_b1933/1 -> Subtract_1dd49/1
  Product_25ba4/1 -> Divide_541d7/1
  Constant_x_l_acc66/1 -> Subtract_1dd49/2
  Divide_01188/1 -> Add_4d303/1
  Product_4d3cc/1 -> Divide_01188/1
  Add_bc191/1 -> Divide_93cdc/2
  Subtract_20a40/1 -> Add_0aa48/1
  Divide_93cdc/1 -> Subtract_20a40/2
  Subtract_32e12/1 -> Divide_30e86/2
  State_psi_fd_SG_D_1_72d5b/1 -> Product_babae/1
  Constant_x_ddd_2cff1/1 -> Divide_541d7/2
  Subtract_1dd49/1 -> Product_babae/2
  Constant_x_dd_3564b/1 -> Subtract_54444/1
  Constant_x_l_921cd/1 -> Subtract_54444/2
  Divide_30e86/1 -> Add_340b6/1
  Add_340b6/1 -> Subtract_aea2e/1
  State_psi_d_SG_D_1_deb78/1 -> Add_340b6/2
  Product_babae/1 -> Divide_ed81b/1
  Subtract_54444/1 -> Divide_ed81b/2
  Constant_-1_170f2/1 -> Product_ad06a/1
  State_psi_d_SG_D_1_175f2/1 -> Product_ad06a/2
  Divide_ed81b/1 -> Subtract_aea2e/2
  Add_0aa48/1 -> Product_4d3cc/2
  Divide_541d7/1 -> Add_4d303/2
  Add_4d303/1 -> Blockout_T_e_SG_D_1_032d2/1

== system case2/SG_D_1/d_E_fd_SG_D_1_block ==
  note: d_E_fd_SG_D_1 in case2
      | $\frac{V_{f,\mathrm{SG},D,1}-E_{\mathrm{fd},\mathrm{SG},D,1}\,K_{E}}{T_{E}}$
      | Automatically generated on 2025-10-31 18:53:41 .
  State_E_fd_SG_D_1_3ff58 : Inport
  State_V_f_SG_D_1_bbd90 : Inport  Port=2
  Add_41ee8 : Sum
  Constant_-1_56d6d : Constant  Value=-1
  Constant_K_E_ff81c : Constant  Value=K_E
  Constant_T_E_ecc04 : Constant  Value=T_E
  Divide_9d198 : Product  Inputs=*/
  Product_01204 : Product
  Product_b2d16 : Product
  Blockout_d_E_fd_SG_D_1_236a3 : Outport
  wires:
  Add_41ee8/1 -> Divide_9d198/1
  Constant_-1_56d6d/1 -> Product_01204/1
  State_E_fd_SG_D_1_3ff58/1 -> Product_01204/2
  Product_01204/1 -> Product_b2d16/1
  Constant_K_E_ff81c/1 -> Product_b2d16/2
  Product_b2d16/1 -> Add_41ee8/1
  Constant_T_E_ecc04/1 -> Divide_9d198/2
  State_V_f_SG_D_1_bbd90/1 -> Add_41ee8/2
  Divide_9d198/1 -> Blockout_d_E_fd_SG_D_1_236a3/1

== system case2/SG_D_1/d_Px_1_SG_D_1_block ==
  note: d_Px_1_SG_D_1 in case2
      | $\frac{w_{\mathrm{SG},D,1}-2\,\pi \,f_{0}}{T_{w}}-\frac{\mathrm{Px}_{1,\mathrm{SG},D,1}}{T_{w}}$
      | Automatically generated on 2025-10-31 18:53:43 .
  State_Px_1_SG_D_1_bfde0 : Inport
  State_w_SG_D_1_30941 : Inport  Port=2
  Add_5b959 : Sum
  Add_999b4 : Sum
  Constant_-1_38359 : Constant  Value=-1
  Constant_-2.0_0a503 : Constant  Value=-2.0
  Constant_T_w_66e46 : Constant  Value=T_w
  Constant_T_w_c47a4 : Constant  Value=T_w
  Constant_f0_b59d9 : Constant  Value=f0
  Constant_pi_5f9a3 : Constant  Value=pi
  Divide_1bc0d : Product  Inputs=*/
  Divide_dfa0e : Product  Inputs=*/
  Product_07155 : Product
  Product_4e089 : Product
  Product_dc245 : Product
  Blockout_d_Px_1_SG_D_1_87980 : Outport
  wires:
  Add_999b4/1 -> Blockout_d_Px_1_SG_D_1_87980/1
  Constant_-2.0_0a503/1 -> Product_4e089/1
  Product_07155/1 -> Divide_dfa0e/1
  State_w_SG_D_1_30941/1 -> Add_5b959/2
  Constant_-1_38359/1 -> Product_07155/1
  Constant_f0_b59d9/1 -> Product_dc245/2
  Constant_pi_5f9a3/1 -> Product_4e089/2
  Product_dc245/1 -> Add_5b959/1
  Product_4e089/1 -> Product_dc245/1
  State_Px_1_SG_D_1_bfde0/1 -> Product_07155/2
  Constant_T_w_c47a4/1 -> Divide_dfa0e/2
  Add_5b959/1 -> Divide_1bc0d/1
  Constant_T_w_66e46/1 -> Divide_1bc0d/2
  Divide_dfa0e/1 -> Add_999b4/1
  Divide_1bc0d/1 -> Add_999b4/2

== system case2/SG_D_1/d_Px_2_SG_D_1_block ==
  note: d_Px_2_SG_D_1 in case2
      | $\frac{\mathrm{Px}_{1,\mathrm{SG},D,1}-T_{2}\,\left(\frac{\mathrm{Px}_{1,\mathrm{SG},D,1}}{T_{w}}-\frac{w_{\mathrm{SG},D,1}-2\,\pi \,f_{0}}{T_{w}}\right)}{T_{1}}-\frac{\mathrm{Px}_{2,\mathrm{SG},D,1}}{T_{1}}$
      | Automatically generated on 2025-10-31 18:53:44 .
  State_Px_2_SG_D_1_f9a06 : Inport
  State_Px_1_SG_D_1_9c7e3 : Inport  Port=2
  State_Px_1_SG_D_1_08e5e : Inport  Port=3
  State_w_SG_D_1_63813 : Inport  Port=4
  Add_3b0ce : Sum
  Add_7c4c9 : Sum
  Add_e5646 : Sum
  Add_fe9c8 : Sum
  Constant_-1_8dd05 : Constant  Value=-1
  Constant_-1_d769a : Constant  Value=-1
  Constant_-2.0_81c1a : Constant  Value=-2.0
  Constant_T_1_3ae30 : Constant  Value=T_1
  Constant_T_1_abcc3 : Constant  Value=T_1
  Constant_T_2_f7b5b : Constant  Value=T_2
  Constant_T_w_187f2 : Constant  Value=T_w
  Constant_T_w_a1960 : Constant  Value=T_w
  Constant_f0_aefca : Constant  Value=f0
  Constant_pi_d3052 : Constant  Value=pi
  Divide_31082 : Product  Inputs=*/
  Divide_9d8f1 : Product  Inputs=*/
  Divide_cae0a : Product  Inputs=*/
  Divide_eb79b : Product  Inputs=*/
  Product_420bd : Product
  Product_8f602 : Product
  Product_ac559 : Product
  Product_bdf3f : Product
  Product_ff209 : Product
  Blockout_d_Px_2_SG_D_1_76795 : Outport
  wires:
  Constant_-2.0_81c1a/1 -> Product_ac559/1
  State_w_SG_D_1_63813/1 -> Add_3b0ce/2
  Constant_f0_aefca/1 -> Product_ff209/2
  Constant_pi_d3052/1 -> Product_ac559/2
  Add_fe9c8/1 -> Product_8f602/2
  Product_ff209/1 -> Add_3b0ce/1
  Divide_cae0a/1 -> Add_fe9c8/1
  Product_ac559/1 -> Product_ff209/1
  Constant_T_w_a1960/1 -> Divide_cae0a/2
  Constant_-1_d769a/1 -> Product_bdf3f/1
  State_Px_1_SG_D_1_08e5e/1 -> Product_bdf3f/2
  Divide_eb79b/1 -> Add_7c4c9/1
  Product_bdf3f/1 -> Divide_cae0a/1
  Add_3b0ce/1 -> Divide_9d8f1/1
  Constant_T_w_187f2/1 -> Divide_9d8f1/2
  Divide_9d8f1/1 -> Add_fe9c8/2
  Constant_T_2_f7b5b/1 -> Product_8f602/1
  Constant_-1_8dd05/1 -> Product_420bd/1
  State_Px_2_SG_D_1_f9a06/1 -> Product_420bd/2
  State_Px_1_SG_D_1_9c7e3/1 -> Add_e5646/1
  Product_8f602/1 -> Add_e5646/2
  Add_e5646/1 -> Divide_31082/1
  Product_420bd/1 -> Divide_eb79b/1
  Constant_T_1_3ae30/1 -> Divide_eb79b/2
  Constant_T_1_abcc3/1 -> Divide_31082/2
  Divide_31082/1 -> Add_7c4c9/2
  Add_7c4c9/1 -> Blockout_d_Px_2_SG_D_1_76795/1

== system case2/SG_D_1/d_Px_3_SG_D_1_block ==
  note: d_Px_3_SG_D_1 in case2
      | $\frac{\mathrm{Px}_{2,\mathrm{SG},D,1}+T_{4}\,\left(\frac{\mathrm{Px}_{1,\mathrm{SG},D,1}-T_{2}\,\left(\frac{\mathrm{Px}_{1,\mathrm{SG},D,1}}{T_{w}}-\frac{w_{\mathrm{SG},D,1}-2\,\pi \,f_{0}}{T_{w}}\right)}{T_{1}}-\frac{\mathrm{Px}_{2,\mathrm{SG},D,1}}{T_{1}}\right)}{T_{3}}-\frac{\mathrm{Px}_{3,\mathrm{SG},D,1}}{T_{3}}$
      | Automatically generated on 2025-10-31 18:53:47 .
  State_Px_3_SG_D_1_70d34 : Inport
  State_Px_2_SG_D_1_26c88 : Inport  Port=2
  State_Px_2_SG_D_1_10f49 : Inport  Port=3
  State_Px_1_SG_D_1_d5924 : Inport  Port=4
  State_Px_1_SG_D_1_8d63f : Inport  Port=5
  State_w_SG_D_1_cb78d : Inport  Port=6
  Add_22a67 : Sum
  Add_46094 : Sum
  Add_9036b : Sum
  Add_99479 : Sum
  Add_b6ba3 : Sum
  Add_dfeca : Sum
  Constant_-1_50311 : Constant  Value=-1
  Constant_-1_bc2d5 : Constant  Value=-1
  Constant_-1_f9436 : Constant  Value=-1
  Constant_-2.0_34655 : Constant  Value=-2.0
  Constant_T_1_4dc67 : Constant  Value=T_1
  Constant_T_1_af88f : Constant  Value=T_1
  Constant_T_2_def9f : Constant  Value=T_2
  Constant_T_3_3f706 : Constant  Value=T_3
  Constant_T_3_45e1e : Constant  Value=T_3
  Constant_T_4_66e6e : Constant  Value=T_4
  Constant_T_w_454bd : Constant  Value=T_w
  Constant_T_w_de2d8 : Constant  Value=T_w
  Constant_f0_81a11 : Constant  Value=f0
  Constant_pi_d80ca : Constant  Value=pi
  Divide_0f860 : Product  Inputs=*/
  Divide_4cc0a : Product  Inputs=*/
  Divide_5a65f : Product  Inputs=*/
  Divide_c1fca : Product  Inputs=*/
  Divide_e7f02 : Product  Inputs=*/
  Divide_f0a0b : Product  Inputs=*/
  Product_447d7 : Product
  Product_47b53 : Product
  Product_7d417 : Product
  Product_88aff : Product
  Product_a5cf9 : Product
  Product_ec879 : Product
  Product_f7c80 : Product
  Blockout_d_Px_3_SG_D_1_a361e : Outport
  wires:
  Constant_T_w_454bd/1 -> Divide_5a65f/2
  Constant_-1_50311/1 -> Product_f7c80/1
  Add_46094/1 -> Blockout_d_Px_3_SG_D_1_a361e/1
  Constant_-2.0_34655/1 -> Product_7d417/1
  State_w_SG_D_1_cb78d/1 -> Add_99479/2
  Constant_f0_81a11/1 -> Product_47b53/2
  State_Px_1_SG_D_1_8d63f/1 -> Product_f7c80/2
  Constant_pi_d80ca/1 -> Product_7d417/2
  Product_47b53/1 -> Add_99479/1
  Product_7d417/1 -> Product_47b53/1
  Product_f7c80/1 -> Divide_5a65f/1
  Divide_c1fca/1 -> Add_46094/1
  Constant_T_3_45e1e/1 -> Divide_f0a0b/2
  Add_99479/1 -> Divide_0f860/1
  Constant_T_w_de2d8/1 -> Divide_0f860/2
  Divide_5a65f/1 -> Add_9036b/1
  Divide_0f860/1 -> Add_9036b/2
  Constant_-1_bc2d5/1 -> Product_ec879/1
  Constant_T_2_def9f/1 -> Product_447d7/1
  Add_9036b/1 -> Product_447d7/2
  Constant_-1_f9436/1 -> Product_a5cf9/1
  Divide_f0a0b/1 -> Add_46094/2
  Constant_T_3_3f706/1 -> Divide_c1fca/2
  State_Px_2_SG_D_1_10f49/1 -> Product_a5cf9/2
  State_Px_1_SG_D_1_d5924/1 -> Add_b6ba3/1
  Divide_4cc0a/1 -> Add_22a67/1
  Product_447d7/1 -> Add_b6ba3/2
  Product_a5cf9/1 -> Divide_4cc0a/1
  Product_ec879/1 -> Divide_c1fca/1
  Constant_T_1_4dc67/1 -> Divide_4cc0a/2
  Add_b6ba3/1 -> Divide_e7f02/1
  Constant_T_1_af88f/1 -> Divide_e7f02/2
  Divide_e7f02/1 -> Add_22a67/2
  Constant_T_4_66e6e/1 -> Product_88aff/1
  Add_22a67/1 -> Product_88aff/2
  State_Px_3_SG_D_1_70d34/1 -> Product_ec879/2
  State_Px_2_SG_D_1_26c88/1 -> Add_dfeca/1
  Product_88aff/1 -> Add_dfeca/2
  Add_dfeca/1 -> Divide_f0a0b/1

== system case2/SG_D_1/d_R_f_SG_D_1_block ==
  note: d_R_f_SG_D_1 in case2
      | $-\frac{R_{f,\mathrm{SG},D,1}-\frac{E_{\mathrm{fd},\mathrm{SG},D,1}\,K_{F}}{T_{F}}}{T_{F}}$
      | Automatically generated on 2025-10-31 18:53:40 .
  State_E_fd_SG_D_1_fbe0c : Inport
  State_R_f_SG_D_1_c3db5 : Inport  Port=2
  Constant_K_F_8b22e : Constant  Value=K_F
  Constant_T_F_1c2ea : Constant  Value=T_F
  Constant_T_F_41c20 : Constant  Value=T_F
  Divide_2a9c3 : Product  Inputs=*/
  Divide_4a2df : Product  Inputs=*/
  Product_cd6eb : Product
  Subtract_b0167 : Sum  Inputs=+-
  Blockout_d_R_f_SG_D_1_43b9e : Outport
  wires:
  Constant_K_F_8b22e/1 -> Product_cd6eb/2
  Product_cd6eb/1 -> Divide_4a2df/1
  State_E_fd_SG_D_1_fbe0c/1 -> Product_cd6eb/1
  State_R_f_SG_D_1_c3db5/1 -> Subtract_b0167/2
  Constant_T_F_1c2ea/1 -> Divide_4a2df/2
  Divide_4a2df/1 -> Subtract_b0167/1
  Divide_2a9c3/1 -> Blockout_d_R_f_SG_D_1_43b9e/1
  Subtract_b0167/1 -> Divide_2a9c3/1
  Constant_T_F_41c20/1 -> Divide_2a9c3/2

== system case2/SG_D_1/d_T_m_SG_D_1_block ==
  note: d_T_m_SG_D_1 in case2
      | $-\frac{T_{m,\mathrm{SG},D,1}-T_{0}+\frac{\mathrm{SpeedPara}\,\left(w_{\mathrm{SG},D,1}-w_{\mathrm{ref}}\right)}{2\,f_{0}\,\pi }}{T_{\mathrm{speed}}}$
      | Automatically generated on 2025-10-31 18:53:31 .
  State_w_SG_D_1_af4aa : Inport
  State_T_m_SG_D_1_b3cab : Inport  Port=2
  Add_37da4 : Sum
  Add_60613 : Sum
  Constant_-1_72e3b : Constant  Value=-1
  Constant_2.0_ac860 : Constant  Value=2.0
  Constant_SpeedPara_5638b : Constant  Value=SpeedPara
  Constant_T_0_3830b : Constant  Value=T_0
  Constant_T_speed_efda0 : Constant  Value=T_speed
  Constant_f0_eaa91 : Constant  Value=f0
  Constant_pi_613d0 : Constant  Value=pi
  Constant_w_ref_0610b : Constant  Value=w_ref
  Divide_5c9bb : Product  Inputs=*/
  Divide_d79be : Product  Inputs=*/
  Product_05644 : Product
  Product_4970b : Product
  Product_67044 : Product
  Product_ee67f : Product
  Subtract_a705e : Sum  Inputs=+-
  Blockout_d_T_m_SG_D_1_1f476 : Outport
  wires:
  Constant_-1_72e3b/1 -> Product_67044/1
  Constant_w_ref_0610b/1 -> Add_60613/2
  State_w_SG_D_1_af4aa/1 -> Product_67044/2
  Add_37da4/1 -> Subtract_a705e/1
  Add_60613/1 -> Product_ee67f/2
  Product_67044/1 -> Add_60613/1
  Constant_2.0_ac860/1 -> Product_05644/1
  Constant_pi_613d0/1 -> Product_05644/2
  Constant_SpeedPara_5638b/1 -> Product_ee67f/1
  Product_05644/1 -> Product_4970b/1
  Constant_f0_eaa91/1 -> Product_4970b/2
  Constant_T_speed_efda0/1 -> Divide_d79be/2
  Product_ee67f/1 -> Divide_5c9bb/1
  Product_4970b/1 -> Divide_5c9bb/2
  Divide_5c9bb/1 -> Add_37da4/1
  Constant_T_0_3830b/1 -> Add_37da4/2
  State_T_m_SG_D_1_b3cab/1 -> Subtract_a705e/2
  Subtract_a705e/1 -> Divide_d79be/1
  Divide_d79be/1 -> Blockout_d_T_m_SG_D_1_1f476/1
